simulink model "AM4"  (R2021a)
settings: Solver=VariableStepAuto  StartTime=0.0  StopTime=10.0  RelTol=1e-3
settings Model: Creator=Devraj Kashyap  LastModifiedBy=Devraj Kashyap

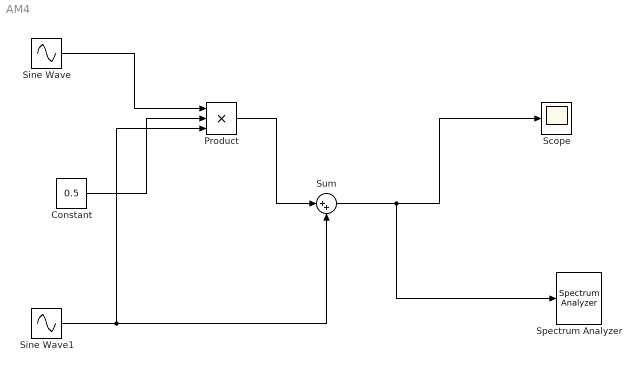
== system AM4 ==
  Constant : Constant  Value=0.5  SampleTime=0.0001
  Product : Product  Inputs=3
  Scope : Scope
  Sine Wave : Sin  Frequency=10  SampleTime=0.0001
  Sine Wave1 : Sin  Frequency=100  Phase=90  SampleTime=0.0001
  Spectrum Analyzer : SpectrumAnalyzer
  Sum : Sum  Inputs=|++
  wires:
  Sine Wave/1 -> Product/1
  Constant/1 -> Product/2
  Sine Wave1/1 -> Sum/2, Product/3
  Product/1 -> Sum/1
  Sum/1 -> Spectrum Analyzer/1, Scope/1
